simulink model "co2_m1"  (R2020a)
settings: Solver=FixedStepAuto  StartTime=0.0  StopTime=20  FixedStep=0.016  RelTol=1e-3
undefined symbols (not defined in the file): alpha, d, phi, tau, tau2
settings Model: Creator=sebastian  LastModifiedBy=sebastian

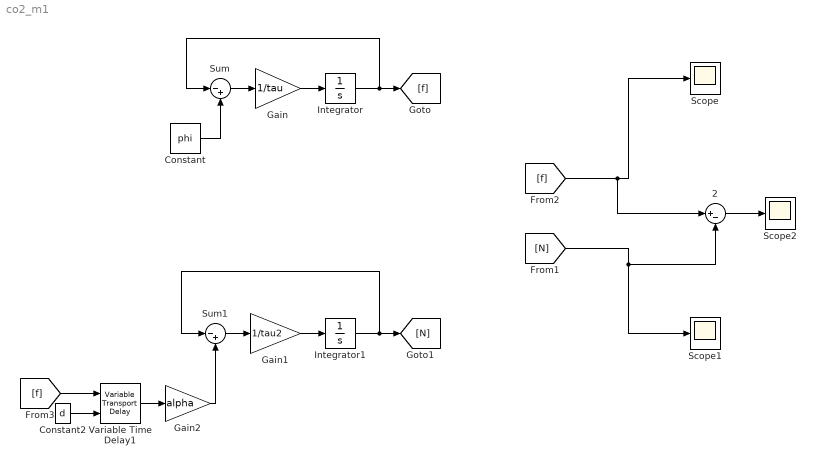
== system co2_m1 ==
  2 : Sum  Inputs=|+-
  Constant : Constant  Value=phi
  Constant2 : Constant  Value=d
  Gain : Gain  Gain=1/tau
  Gain1 : Gain  Gain=1/tau2
  Gain2 : Gain  Gain=alpha
  Integrator : Integrator
  Integrator1 : Integrator
  Scope : Scope
  Scope1 : Scope
  Scope2 : Scope
  Sum : Sum  Inputs=|-+
  Sum1 : Sum  Inputs=|-+
  Variable Time Delay1 : VariableTransportDelay  MaximumDelay=10
  wires:
  Sum/1 -> Gain/1
  Gain/1 -> Integrator/1
  Constant/1 -> Sum/2
  Integrator/1 -> [f], Sum/1
  Gain1/1 -> Integrator1/1
  Sum1/1 -> Gain1/1
  Integrator1/1 -> [N], Sum1/1
  Gain2/1 -> Sum1/2
  [f] -> 2/1, Scope/1
  [N] -> 2/2, Scope1/1
  [f] -> Variable Time Delay1/1
  Constant2/1 -> Variable Time Delay1/2
  Variable Time Delay1/1 -> Gain2/1
  2/1 -> Scope2/1
